simulink model "RIP_Cascade_PID"  (R2022b)
settings: Solver=ode4  StartTime=0.0  StopTime=20  FixedStep=0.001  RelTol=1e-3
undefined symbols (not defined in the file): A, B, C, D, init_alpha, init_alpha_dot, init_theta, init_theta_dot, X_0
libraries: simulink_extras x6, cstblocks x2
settings Model: Creator=Andrew  LastModifiedBy=Andrew

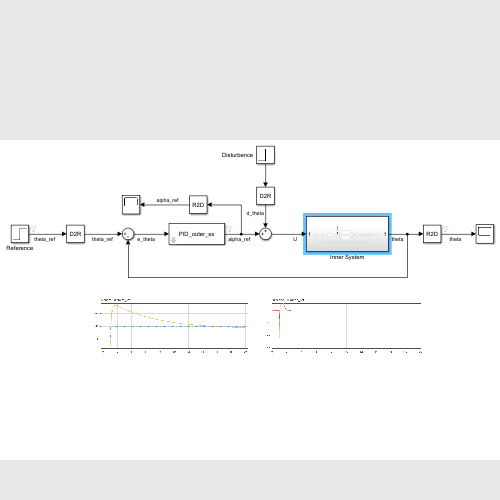
[thumbnail: Simulink's stored preview of the top-level diagram]
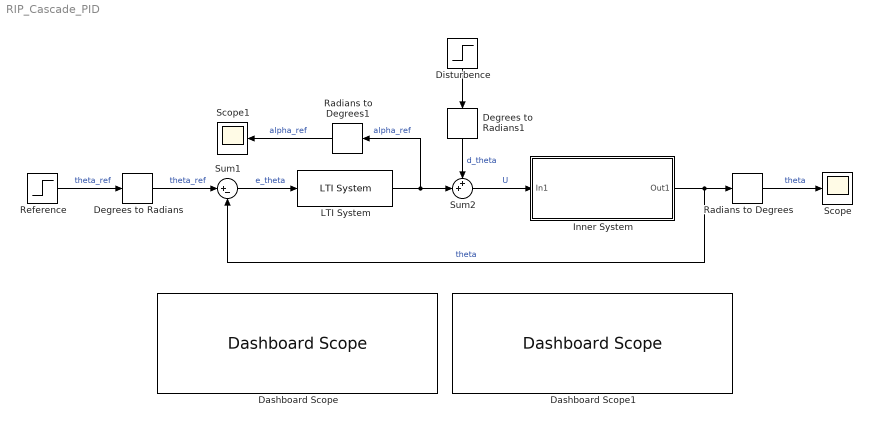
== system RIP_Cascade_PID ==
  Dashboard Scope : DashboardScope  NormalizeYAxis=on
  Dashboard Scope1 : DashboardScope  NormalizeYAxis=on
  Degrees to Radians : simulink_extras/Transformations/Degrees to Radians
  Degrees to Radians1 : simulink_extras/Transformations/Degrees to Radians
  Disturbence : Step  Time=0  After=0  SampleTime=0
  Inner System : Subsystem
  LTI System : cstblocks/LTI System  sys=PID_outer_ss  IC=[]
  Radians to Degrees : simulink_extras/Transformations/Radians to Degrees
  Radians to Degrees1 : simulink_extras/Transformations/Radians to Degrees
  Reference : Step  After=50  SampleTime=0
  Scope : Scope
  Scope1 : Scope
  Sum1 : Sum  Inputs=|+-
  Sum2 : Sum  Inputs=++|
  wires:
  Radians to Degrees/1 -> Scope/1  "theta"
  Degrees to Radians1/1 -> Sum2/1  "d_theta"
  Disturbence/1 -> Degrees to Radians1/1
  Inner System/1(Out1) -> Sum1/2, Radians to Degrees/1  "theta"
  Reference/1 -> Degrees to Radians/1  "theta_ref"
  Degrees to Radians/1 -> Sum1/1  "theta_ref"
  Sum2/1 -> Inner System/1(In1)  "U"
  Sum1/1 -> LTI System/1  "e_theta"
  LTI System/1 -> Radians to Degrees1/1, Sum2/2  "alpha_ref"
  Radians to Degrees1/1 -> Scope1/1  "alpha_ref"

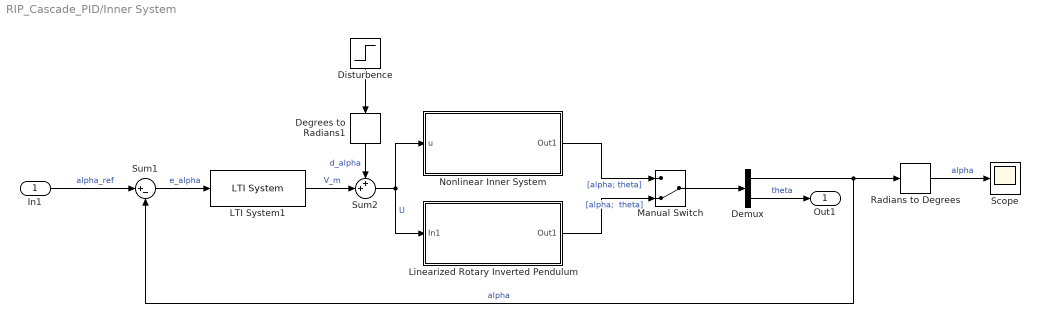
== system RIP_Cascade_PID/Inner System ==
  In1 : Inport
  Degrees to Radians1 : simulink_extras/Transformations/Degrees to Radians
  Demux : Demux  Outputs=2
  Disturbence : Step  Time=0  After=0  SampleTime=0
  LTI System1 : cstblocks/LTI System  sys=PID_alpha_ss  IC=[]
  Linearized Rotary Inverted Pendulum : Subsystem  Tag=SISO_alpha
  Manual Switch : ManualSwitch  CurrentSetting=0
  Nonlinear Inner System : Subsystem
  Radians to Degrees : simulink_extras/Transformations/Radians to Degrees
  Scope : Scope
  Sum1 : Sum  Inputs=|+-
  Sum2 : Sum  Inputs=++|
  Out1 : Outport
  wires:
  Degrees to Radians1/1 -> Sum2/1  "d_alpha"
  Disturbence/1 -> Degrees to Radians1/1
  Demux/2 -> Out1/1  "theta"
  Demux/1 -> Radians to Degrees/1, Sum1/2  "alpha"
  In1/1 -> Sum1/1  "alpha_ref"
  Sum1/1 -> LTI System1/1  "e_alpha"
  LTI System1/1 -> Sum2/2  "V_m"
  Sum2/1 -> Nonlinear Inner System/1(u), Linearized Rotary Inverted Pendulum/1(In1)  "U"
  Nonlinear Inner System/1(Out1) -> Manual Switch/1  "[alpha; theta]"
  Linearized Rotary Inverted Pendulum/1(Out1) -> Manual Switch/2  "[alpha;  theta]"
  Manual Switch/1 -> Demux/1
  Radians to Degrees/1 -> Scope/1  "alpha"

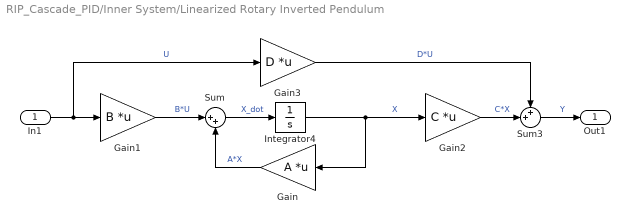
== system RIP_Cascade_PID/Inner System/Linearized Rotary Inverted Pendulum ==
  In1 : Inport
  Gain : Gain  Gain=A  Multiplication=Matrix(K*u) (u vector)
  Gain1 : Gain  Gain=B  Multiplication=Matrix(K*u) (u vector)
  Gain2 : Gain  Gain=C  Multiplication=Matrix(K*u) (u vector)
  Gain3 : Gain  Gain=D  Multiplication=Matrix(K*u) (u vector)
  Integrator4 : Integrator  InitialCondition=[init_alpha; init_alpha_dot; init_theta; init_theta_dot]
  Sum : Sum  Inputs=|++
  Sum3 : Sum  Inputs=++|
  Out1 : Outport
  wires:
  Gain2/1 -> Sum3/2  "C*X"
  Gain/1 -> Sum/2  "A*X"
  Gain3/1 -> Sum3/1  "D*U"
  Gain1/1 -> Sum/1  "B*U"
  Sum/1 -> Integrator4/1  "X_dot"
  Integrator4/1 -> Gain2/1, Gain/1  "X"
  In1/1 -> Gain3/1, Gain1/1  "U"
  Sum3/1 -> Out1/1  "Y"

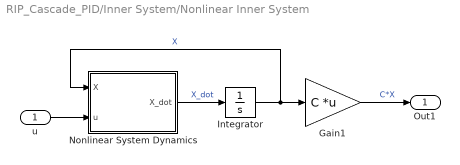
== system RIP_Cascade_PID/Inner System/Nonlinear Inner System ==
  u : Inport
  Gain1 : Gain  Gain=C  Multiplication=Matrix(K*u) (u vector)
  Integrator : Integrator  InitialCondition=X_0
  Nonlinear System Dynamics : MATLAB Function  TreatAsAtomicUnit=on
  Out1 : Outport
  wires:
  Nonlinear System Dynamics/1(X_dot) -> Integrator/1  "X_dot"
  Integrator/1 -> Gain1/1, Nonlinear System Dynamics/1(X)  "X"
  u/1 -> Nonlinear System Dynamics/2(u)
  Gain1/1 -> Out1/1  "C*X"

== matlab function RIP_Cascade_PID/Inner System/Nonlinear Inner System/Nonlinear System Dynamics ==
  data: X input; u input; X_dot output
function X_dot = fcn(X, u)


x_1 = X(1);           % Alpha
x_2 = X(2);           % Alpha_dot
x_3 = X(3);           % Theta (Doesnt directly play role in the system dynamics)
x_4 = X(4);           % Theta_dot

g = 9.83;             % Gravitational acceleration (m/s^2)

% Rotary Inverted Pendulum Parameters 
m_p = 0.127;          % Mass of pendulum (kg)
L_p = 0.337;          % Total length of pendulum (m)
L_r = 0.216;          % Rotary arm length from pivot to tip (m)
J_p = 0.0012;         % Pendulum moment of inertia about center of mass (kg.m^2)
J_r = 0.0020 ;        % Rotary arm moment of inertia about center of mass (kg.m^2)
B_p = 0.0024;         % Pendulum viscous damping coefficient (N.m.s/rad)
B_r = 0.0024;         % Rotary arm viscous damping coefficient (N.m.s/rad)

% Rotary Servo Base Unit Parameters 
R_m = 2.6;            % Motor armature resistance (ohms)
k_t = 7.68e-3;        % Motor current-torque constant (N.m/A)
k_m = 7.68e-3;        % Motor back-emf constant (V/(rad/s))
K_g = 70;             % High-gear total gear ratio [-]
eta_m = 0.69;         % Motor efficiency [-]
eta_g = 0.90;         % Gearbox efficiency [-]

x_dot_1 = x_2;
x_dot_2 = -(8*eta_g*eta_m*k_m*k_t*K_g^2*L_p*L_r*m_p*x_4*cos(x_1) - 8*eta_g*eta_m*k_t*u*K_g*L_p*L_r*m_p*cos(x_1) + R_m*sin(x_1)*L_p^4*m_p^2*x_4^2*cos(x_1)^3 - R_m*sin(x_1)*L_p^4*m_p^2*x_4^2*cos(x_1) + 4*R_m*sin(x_1)*L_p^3*L_r*m_p^2*x_2*x_4*cos(x_1)^2 + 2*R_m*g*sin(x_1)*L_p^3*m_p^2*cos(x_1)^2 - 2*R_m*g*sin(x_1)*L_p^3*m_p^2 + 4*R_m*sin(x_1)*L_p^2*L_r^2*m_p^2*x_2^2*cos(x_1) - 4*R_m*sin(x_1)*L_p^2*L_r^2*m_p^2*x_4^2*cos(x_1) - 4*B_p*R_m*L_p^2*m_p*x_2*cos(x_1)^2 + 4*B_p*R_m*L_p^2*m_p*x_2 - 4*J_r*R_m*sin(x_1)*L_p^2*m_p*x_4^2*cos(x_1) - 8*R_m*g*sin(x_1)*L_p*L_r^2*m_p^2 + 8*B_r*R_m*L_p*L_r*m_p*x_4*cos(x_1) - 8*J_r*R_m*g*sin(x_1)*L_p*m_p + 16*B_p*R_m*L_r^2*m_p*x_2 + 16*B_p*J_r*R_m*x_2)/(R_m*(L_p^4*m_p^2 + 16*J_p*J_r - L_p^4*m_p^2*cos(x_1)^2 + 4*L_p^2*L_r^2*m_p^2 + 4*J_p*L_p^2*m_p + 16*J_p*L_r^2*m_p + 4*J_r*L_p^2*m_p - 4*L_p^2*L_r^2*m_p^2*cos(x_1)^2 - 4*J_p*L_p^2*m_p*cos(x_1)^2));
x_dot_3 = x_4;
x_dot_4 = -(2*(2*eta_g*eta_m*k_m*k_t*K_g^2*L_p^2*m_p*x_4 + 8*J_p*eta_g*eta_m*k_m*k_t*K_g^2*x_4 - 2*eta_g*eta_m*k_t*u*K_g*L_p^2*m_p - 8*J_p*eta_g*eta_m*k_t*u*K_g + R_m*sin(x_1)*L_p^4*m_p^2*x_2*x_4*cos(x_1) + L_r*R_m*sin(x_1)*L_p^3*m_p^2*x_2^2 - L_r*R_m*sin(x_1)*L_p^3*m_p^2*x_4^2*cos(x_1)^2 - 2*L_r*R_m*g*sin(x_1)*L_p^2*m_p^2*cos(x_1) + 4*J_p*R_m*sin(x_1)*L_p^2*m_p*x_2*x_4*cos(x_1) + 2*B_r*R_m*L_p^2*m_p*x_4 + 4*J_p*L_r*R_m*sin(x_1)*L_p*m_p*x_2^2 + 4*B_p*L_r*R_m*L_p*m_p*x_2*cos(x_1) + 8*B_r*J_p*R_m*x_4))/(R_m*(L_p^4*m_p^2 + 16*J_p*J_r - L_p^4*m_p^2*cos(x_1)^2 + 4*L_p^2*L_r^2*m_p^2 + 4*J_p*L_p^2*m_p + 16*J_p*L_r^2*m_p + 4*J_r*L_p^2*m_p - 4*L_p^2*L_r^2*m_p^2*cos(x_1)^2 - 4*J_p*L_p^2*m_p*cos(x_1)^2));

X_dot = [x_dot_1; x_dot_2; x_dot_3; x_dot_4];
